simulink model "Sim_1D"  (R2021b)
settings: Solver=FixedStepAuto  StartTime=0.0  FixedStep=0.0001  RelTol=1e-3
values from neighbouring files (symbols this model uses):
  Cx = 0.47    [Final.m]
  g = 9.81    [Final.m]
  J3 = J4 + Jbell    (= 9.15416666667e-06)    [Final.m]
  J4 = m4*a4^2/12    (= 6.3375e-06)    [Final.m]
  k_sol = 100    [Final.m]
  k_sol_vit = 10    [Final.m]
  kc3 = mean(C3(2:end)/w3(2:end).^2)    [Final.m]
  kc4 = mean(C4(2:end)/w4(2:end).^2)    [Final.m]
  kf3 = mean(F3/w3.^2)    [Final.m]
  kf4 = mean(F4/w4.^2)    [Final.m]
  ki3 = kv3    [Final.m]
  ki4 = kv4    [Final.m]
  kv3 = mean((U3-R3*I3)/w3)    [Final.m]
  kv4 = mean((U4-R4*I4)/w4)    [Final.m]
  m = 0.040    (= 0.04)    [Final.m]
  R3 = 4.6    [Final.m]
  R4 = 4.6    [Final.m]
  rho = 1.2    [Final.m]
  S_front = pi*(D_front/2)^2    (= 0.000907920276887)    [Final.m]
  z0 = 0    [Final.m]
  z0_p = 0    [Final.m]
  z_g = 3e-2    (= 0.03)    [Final.m]
libraries: slpidlib x1
settings Model: Creator=laborie30  LastModifiedBy=amblard9
settings DataIOCC: ReturnWorkspaceOutputs=off

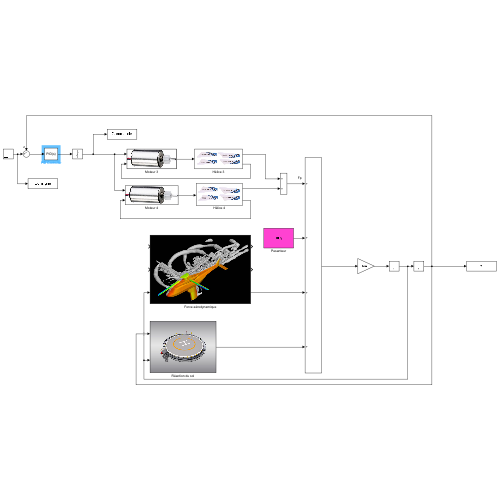
[thumbnail: Simulink's stored preview of the top-level diagram]
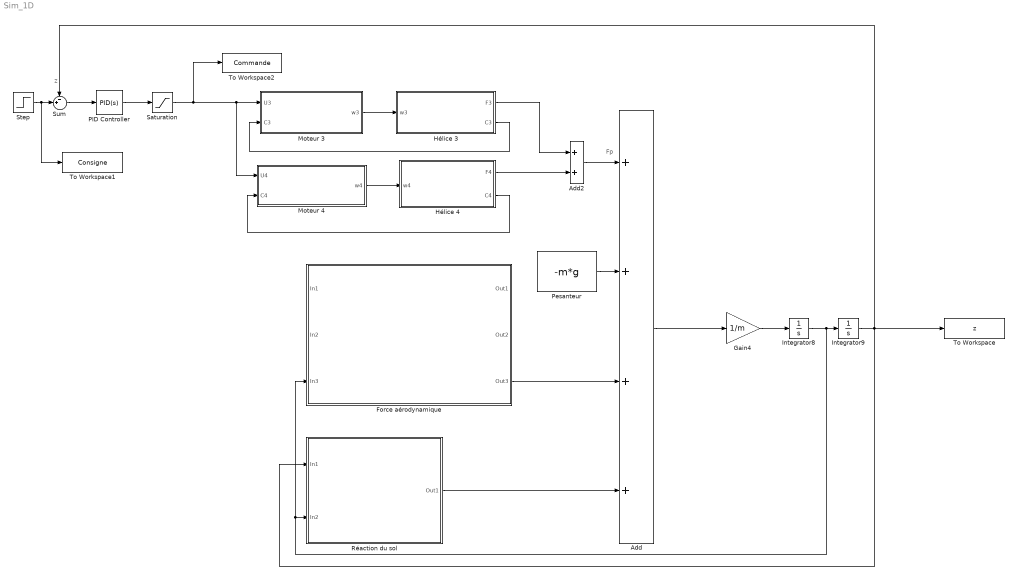
== system Sim_1D ==
  note: Fp
  note: z
  Add : Sum  Inputs=++++
  Add2 : Sum
  Force aérodynamique : Subsystem
      mask Display: image('$imagefile'); % Use "Edit Image" on toolstrip to change.
  Gain4 : Gain  Gain=1/m
  Hélice 3 : Subsystem
      mask Display: image('$imagefile'); % Use "Edit Image" on toolstrip to change.
  Hélice 4 : Subsystem
      mask Display: image('$imagefile'); % Use "Edit Image" on toolstrip to change.
  Integrator8 : Integrator  InitialCondition=z0_p
  Integrator9 : Integrator  InitialCondition=z0
  Moteur 3 : Subsystem
      mask Display: image('$imagefile'); % Use "Edit Image" on toolstrip to change.
  Moteur 4 : Subsystem
      mask Display: image('$imagefile'); % Use "Edit Image" on toolstrip to change.
  PID Controller : slpidlib/PID Controller  Controller=PID  Form=Parallel  TimeDomain=Continuous-time  UseExternalTs=off  SampleTime=-1  IntegratorMethod=Forward Euler  FilterMethod=Forward Euler  ControllerParametersSource=internal  P=7  I=5  D=4  UseFilter=on  N=100  TunerSelectOption=Transfer Function Based (PID Tuner App)  InitialConditionSource=internal  InitialConditionForIntegrator=0  InitialConditionForFilter=0  DifferentiatorICPrevScaledInput=0  ExternalReset=none  TrackingMode=off  Kt=1  LimitOutput=off  SatLimitsSource=internal  UpperSaturationLimit=inf  LowerSaturationLimit=-inf  LinearizeAsGain=on  AntiWindupMode=none  Kb=1  POutMin=[]  POutMax=[]  IOutMin=[]  IOutMax=[]  DOutMin=[]  DOutMax=[]  NOutMin=[]  NOutMax=[]  SumOutMin=[]  SumOutMax=[]  SaturationOutMin=[]  SaturationOutMax=[]  PParamMin=[]  PParamMax=[]  IParamMin=[]  IParamMax=[]  DParamMin=[]  DParamMax=[]  NParamMin=[]  NParamMax=[]  KbParamMin=[]  KbParamMax=[]  KtParamMin=[]  KtParamMax=[]  KbOutMin=[]  KbOutMax=[]  KtOutMin=[]  KtOutMax=[]  IntegratorOutMin=[]  IntegratorOutMax=[]  FilterOutMin=[]  FilterOutMax=[]  SumI1OutMin=[]  SumI1OutMax=[]  SumI2OutMin=[]  SumI2OutMax=[]  SumI3OutMin=[]  SumI3OutMax=[]  SumI4OutMin=[]  SumI4OutMax=[]  SumDOutMin=[]  SumDOutMax=[]  DifferentiatorOutMin=[]  DifferentiatorOutMax=[]  FilterDiffOutCoefMin=[]  FilterDiffOutCoefMax=[]  ReciprocalOutMin=[]  ReciprocalOutMax=[]  SumDenOutMin=[]  SumDenOutMax=[]  SumNumOutMin=[]  SumNumOutMax=[]  DivideOutMin=[]  DivideOutMax=[]  UdiffTsProdOutMin=[]  UdiffTsProdOutMax=[]  NTsProdOutMin=[]  NTsProdOutMax=[]  UintegralTsProdOutMin=[]  UintegralTsProdOutMax=[]  UngainTsProdOutMin=[]  UngainTsProdOutMax=[]  IntegratorContinuousStateAttributes=''  IntegratorStateMustResolveToSignalObject=off  IntegratorRTWStateStorageClass=Auto  FilterContinuousStateAttributes=''  FilterStateMustResolveToSignalObject=off  FilterRTWStateStorageClass=Auto  ParallelPVariant=InternalParameters  IdealPVariant=Disabled  IVariant=InternalParameters  DVariant=InternalParameters  IntegratorVariant=Continuous  SatVariant=Disabled  AWVariant=Passthrough  PCopyVariant=Disabled  TRVariant=Disabled  FdbkBlocksVariant=Forward  IdealPFdbkVariant=Disabled  SatFdbkVariant=Disabled  DerivativeFilterVariant=ContFilter  NVariant=InternalParameters  NCopyVariant=Disabled  FilterICVariant=InternalICsFilter  IntegratorICVariant=InternalICs  ExternalResetVariant=Disabled  TRSumVariant=Passthrough  SumFdbkVariant=Disabled  SumVariant=Sum_PID  TsampFilterVariant=InternalTs  TsampNgainVariant=Passthrough  TsampIntegralVariant=Passthrough  ExternalSaturationOutDataTypeStr=Inherit: Same as second input
  Pesanteur : Constant  Value=-m*g
  Réaction du sol : Subsystem
      mask Display: image('$imagefile'); % Use "Edit Image" on toolstrip to change.
  Saturation : Saturate  UpperLimit=10  LowerLimit=-10
  Step : Step  SampleTime=0
  Sum : Sum  Inputs=-+|
  To Workspace : ToWorkspace  VariableName=z  SampleTime=-1
  To Workspace1 : ToWorkspace  VariableName=Consigne  SampleTime=-1
  To Workspace2 : ToWorkspace  VariableName=Commande  SampleTime=-1
  wires:
  Integrator8/1 -> Réaction du sol/2(In2), Force aérodynamique/3(In3), Integrator9/1
  Gain4/1 -> Integrator8/1
  Add/1 -> Gain4/1
  Hélice 3/2(C3) -> Moteur 3/2(C3)
  Moteur 3/1(w3) -> Hélice 3/1(w3)
  Hélice 4/1(F4) -> Add2/2
  Hélice 3/1(F3) -> Add2/1
  Hélice 4/2(C4) -> Moteur 4/2(C4)
  Moteur 4/1(w4) -> Hélice 4/1(w4)
  Integrator9/1 -> Sum/1, Réaction du sol/1(In1), To Workspace/1
  PID Controller/1 -> Saturation/1
  Sum/1 -> PID Controller/1
  Saturation/1 -> To Workspace2/1, Moteur 4/1(U4), Moteur 3/1(U3)
  Add2/1 -> Add/1
  Réaction du sol/1(Out1) -> Add/4
  Force aérodynamique/3(Out3) -> Add/3
  Pesanteur/1 -> Add/2
  Step/1 -> To Workspace1/1, Sum/2

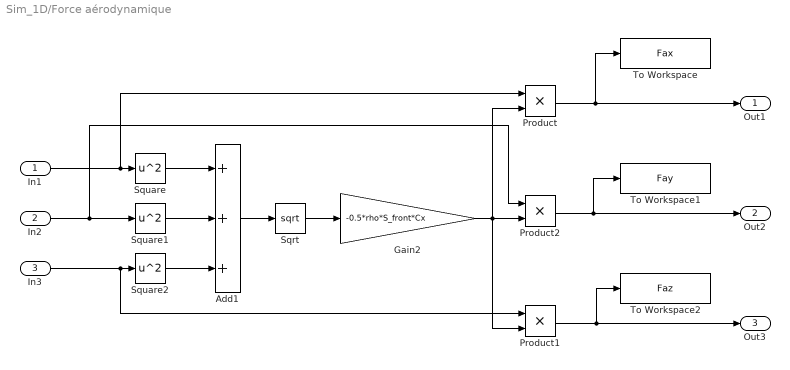
== system Sim_1D/Force aérodynamique ==
  In1 : Inport
  In2 : Inport  Port=2
  In3 : Inport  Port=3
  Add1 : Sum  Inputs=+++
  Gain2 : Gain  Gain=-0.5*rho*S_front*Cx
  Product : Product
  Product1 : Product
  Product2 : Product
  Sqrt : Sqrt  SaturateOnIntegerOverflow=on
  Square : Math  Operator=square  SaturateOnIntegerOverflow=on
  Square1 : Math  Operator=square  SaturateOnIntegerOverflow=on
  Square2 : Math  Operator=square  SaturateOnIntegerOverflow=on
  To Workspace : ToWorkspace  VariableName=Fax  SampleTime=-1
  To Workspace1 : ToWorkspace  VariableName=Fay  SampleTime=-1
  To Workspace2 : ToWorkspace  VariableName=Faz  SampleTime=-1
  Out1 : Outport
  Out2 : Outport  Port=2
  Out3 : Outport  Port=3
  wires:
  In1/1 -> Product/1, Square/1
  Square2/1 -> Add1/3
  In3/1 -> Square2/1, Product1/1
  Gain2/1 -> Product1/2, Product/2, Product2/2
  Sqrt/1 -> Gain2/1
  Add1/1 -> Sqrt/1
  Square/1 -> Add1/1
  Product2/1 -> Out2/1, To Workspace1/1
  Square1/1 -> Add1/2
  In2/1 -> Product2/1, Square1/1
  Product/1 -> Out1/1, To Workspace/1
  Product1/1 -> Out3/1, To Workspace2/1

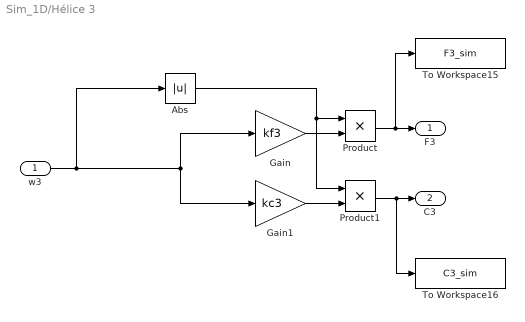
== system Sim_1D/Hélice 3 ==
  w3 : Inport
  Abs : Abs
  Gain : Gain  Gain=kf3
  Gain1 : Gain  Gain=kc3
  Product : Product
  Product1 : Product
  To Workspace15 : ToWorkspace  VariableName=F3_sim  SampleTime=-1
  To Workspace16 : ToWorkspace  VariableName=C3_sim  SampleTime=-1
  F3 : Outport  Unit=N
  C3 : Outport  Port=2  Unit=N*m
  wires:
  w3/1 -> Gain/1, Gain1/1, Abs/1
  Abs/1 -> Product1/1, Product/1
  Product/1 -> To Workspace15/1, F3/1
  Gain/1 -> Product/2
  Gain1/1 -> Product1/2
  Product1/1 -> To Workspace16/1, C3/1

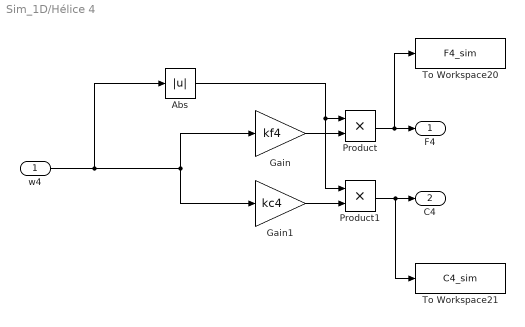
== system Sim_1D/Hélice 4 ==
  w4 : Inport
  Abs : Abs
  Gain : Gain  Gain=kf4
  Gain1 : Gain  Gain=kc4
  Product : Product
  Product1 : Product
  To Workspace20 : ToWorkspace  VariableName=F4_sim  SampleTime=-1
  To Workspace21 : ToWorkspace  VariableName=C4_sim  SampleTime=-1
  F4 : Outport  Unit=N
  C4 : Outport  Port=2  Unit=N*m
  wires:
  w4/1 -> Abs/1, Gain/1, Gain1/1
  Product/1 -> To Workspace20/1, F4/1
  Gain/1 -> Product/2
  Gain1/1 -> Product1/2
  Product1/1 -> To Workspace21/1, C4/1
  Abs/1 -> Product1/1, Product/1

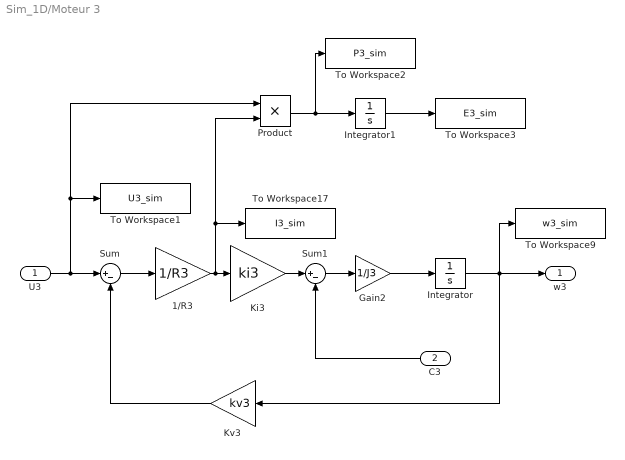
== system Sim_1D/Moteur 3 ==
  U3 : Inport
  C3 : Inport  Port=2
  1/R3 : Gain  Gain=1/R3
  Gain2 : Gain  Gain=1/J3
  Integrator : Integrator
  Integrator1 : Integrator
  Ki3 : Gain  Gain=ki3
  Kv3 : Gain  Gain=kv3
  Product : Product
  Sum : Sum  Inputs=|+-
  Sum1 : Sum  Inputs=|+-
  To Workspace1 : ToWorkspace  VariableName=U3_sim  SampleTime=-1
  To Workspace17 : ToWorkspace  VariableName=I3_sim  SampleTime=-1
  To Workspace2 : ToWorkspace  VariableName=P3_sim  SampleTime=-1
  To Workspace3 : ToWorkspace  VariableName=E3_sim  SampleTime=-1
  To Workspace9 : ToWorkspace  VariableName=w3_sim  SampleTime=-1
  w3 : Outport
  wires:
  Sum/1 -> 1/R3/1
  Kv3/1 -> Sum/2
  Integrator/1 -> Kv3/1, To Workspace9/1, w3/1
  Ki3/1 -> Sum1/1
  1/R3/1 -> Product/2, To Workspace17/1, Ki3/1
  U3/1 -> Product/1, To Workspace1/1, Sum/1
  Sum1/1 -> Gain2/1
  Gain2/1 -> Integrator/1
  C3/1 -> Sum1/2
  Product/1 -> To Workspace2/1, Integrator1/1
  Integrator1/1 -> To Workspace3/1

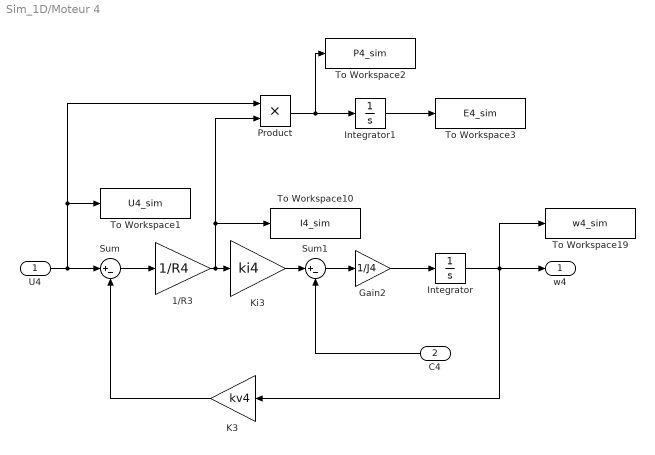
== system Sim_1D/Moteur 4 ==
  U4 : Inport
  C4 : Inport  Port=2
  1/R3 : Gain  Gain=1/R4
  Gain2 : Gain  Gain=1/J4
  Integrator : Integrator
  Integrator1 : Integrator
  K3 : Gain  Gain=kv4
  Ki3 : Gain  Gain=ki4
  Product : Product
  Sum : Sum  Inputs=|+-
  Sum1 : Sum  Inputs=|+-
  To Workspace1 : ToWorkspace  VariableName=U4_sim  SampleTime=-1
  To Workspace10 : ToWorkspace  VariableName=I4_sim  SampleTime=-1
  To Workspace19 : ToWorkspace  VariableName=w4_sim  SampleTime=-1
  To Workspace2 : ToWorkspace  VariableName=P4_sim  SampleTime=-1
  To Workspace3 : ToWorkspace  VariableName=E4_sim  SampleTime=-1
  w4 : Outport
  wires:
  Sum/1 -> 1/R3/1
  K3/1 -> Sum/2
  Integrator/1 -> K3/1, To Workspace19/1, w4/1
  Ki3/1 -> Sum1/1
  Sum1/1 -> Gain2/1
  Gain2/1 -> Integrator/1
  C4/1 -> Sum1/2
  U4/1 -> Product/1, To Workspace1/1, Sum/1
  Integrator1/1 -> To Workspace3/1
  1/R3/1 -> Product/2, To Workspace10/1, Ki3/1
  Product/1 -> To Workspace2/1, Integrator1/1

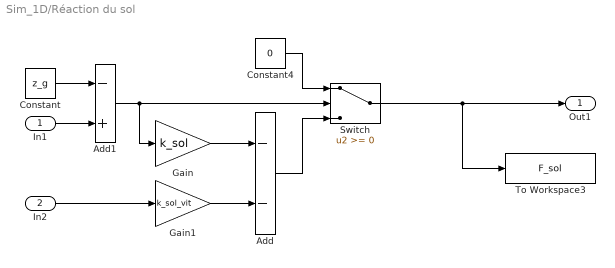
== system Sim_1D/Réaction du sol ==
  In1 : Inport
  In2 : Inport  Port=2
  Add : Sum  Inputs=--
  Add1 : Sum  Inputs=-+
  Constant : Constant  Value=z_g
  Constant4 : Constant  Value=0
  Gain : Gain  Gain=k_sol
  Gain1 : Gain  Gain=k_sol_vit
  Switch : Switch
  To Workspace3 : ToWorkspace  VariableName=F_sol  SampleTime=-1
  Out1 : Outport
  wires:
  Add/1 -> Switch/3
  Gain1/1 -> Add/2
  In2/1 -> Gain1/1
  Gain/1 -> Add/1
  Switch/1 -> Out1/1, To Workspace3/1
  Constant4/1 -> Switch/1
  Add1/1 -> Gain/1, Switch/2
  In1/1 -> Add1/2
  Constant/1 -> Add1/1
